simulink model "MA4EE311Simu_2"  (R2019b)
settings: Solver=VariableStepAuto  StartTime=0.0  StopTime=5  RelTol=1e-3
libraries: dspsnks4 x1, dspsrcs4 x1
settings Model: Creator=hp  LastModifiedBy=hp

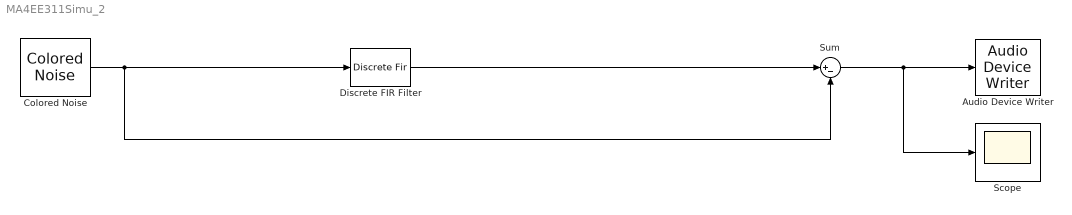
== system MA4EE311Simu_2 ==
  Audio Device Writer : dspsnks4/Audio Device Writer  Driver=DirectSound  Device=Default  InheritSampleRate=on  SampleRate=44100  BitDepth=16-bit integer  BufferSize=4096  NumBuffers=10  DefaultOutputChannelMapping=on  OutputChannelMapping=1:2  OutputNumUnderrunSamples=off  DriverIdx=1  DeviceWarnFlag=''
  Colored Noise : dspsrcs4/Colored Noise  Color=pink  InverseFrequencyPower=1  BoundedOutput=off  NumChannels=1  OutputDataType=double  SamplesPerFrame=1  SampleTime=1/8000  RandomStream=mt19937ar with seed  Seed=67  SimulateUsing=Interpreted execution
      settings: SourceProductName=DSP System Toolbox  SourceProductBaseCode=DS
  Discrete FIR Filter : DiscreteFir  Coefficients=[0.5 0.1 0.2 0.4 0 0 -0.125 0.3 0.5 0 0.075 -0.25 -0.4]  InputProcessing=Columns as channels (frame based)
  Scope : Scope
  Sum : Sum  Inputs=|+-
  wires:
  Colored Noise/1 -> Discrete FIR Filter/1, Sum/2
  Sum/1 -> Scope/1, Audio Device Writer/1
  Discrete FIR Filter/1 -> Sum/1
